simulink model "Automatisierung_Kapitel8_zustandsregler"  (R2015b)
settings: Solver=ode45  StartTime=0.0  StopTime=100  MaxStep=0.2  RelTol=1e-3
values from neighbouring files (symbols this model uses):
  Ac = [0,1,0,0;-1,-1,1,1;0,0,0,1;0.1,0.1,-0.2,-0.2]    [Automatisierung_Kapitel8.m]
  Bc = [bc,bvc]    [Automatisierung_Kapitel8.m]
  Cc = eye(4)    [Automatisierung_Kapitel8.m]
  Dc = [0,0;0,0;0,0;0,0]    [Automatisierung_Kapitel8.m]
  g = 1/((cc+dc*k)*inv(eye(4)-Ad-bd*k)*bd+dc)    [Automatisierung_Kapitel8.m]
  k = -acker(Ad,bd,pd)    [Automatisierung_Kapitel8.m]
  Ta = 2    [Automatisierung_Kapitel8.m]
settings Model: Creator=aku  LastModifiedBy=hk
settings DataIOCC: SaveFormat=Array  SignalLoggingSaveFormat=ModelDataLogs
settings OptimizationCC: BooleanDataType=off  ExpressionDepthLimit=2147483647  InitFltsAndDblsToZero=on
settings DebuggingCC: SaveWithParameterizedLinksMsg=none  UnderspecifiedInitializationDetection=Classic  MergeDetectMultiDrivingBlocksExec=none  SignalResolutionControl=TryResolveAllWithWarning  MultiTaskDSMMsg=warning  MultiTaskCondExecSysMsg=none  FcnCallInpInsideContextMsg=EnableAllAsWarning  StateNameClashWarn=warning
settings HardwareCC: ProdBitPerPointer=32  ProdLargestAtomicFloat=None  ProdIntDivRoundTo=Undefined  ProdEndianess=Unspecified  ProdWordSize=32  ProdHWDeviceType=32-bit Generic  TargetUnknown=on
settings GRTTargetCC: TargetFcnLib=ansi_tfl_tmw.mat  GeneratePreprocessorConditionals=Disable all  CombineOutputUpdateFcns=off  GRTInterface=on
settings ConfigComp: CovModelRefEnable=Off  CovSFcnEnable=off

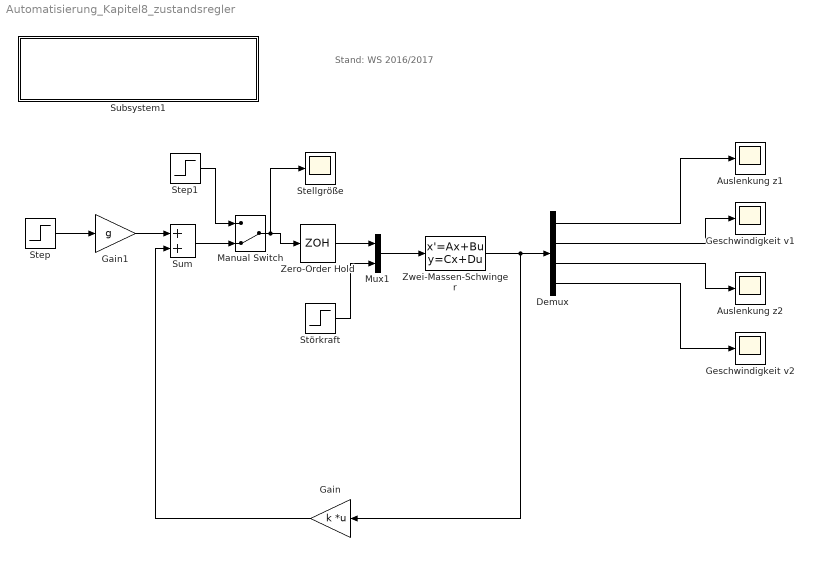
== system Automatisierung_Kapitel8_zustandsregler ==
  note: Stand: WS 2016/2017
  Auslenkung z1 : Scope
  Auslenkung z2 : Scope
  Demux : Demux
  Gain : Gain  Gain=k  Multiplication=Matrix(K*u)  SampleTime=Ta
  Gain1 : Gain  Gain=g  SampleTime=Ta
  Geschwindigkeit v1 : Scope
  Geschwindigkeit v2 : Scope
  Manual Switch : ManualSwitch  CurrentSetting=0
  Mux1 : Mux  Inputs=2
  Stellgröße : Scope
  Step : Step  Time=0  SampleTime=Ta
  Step1 : Step  Time=0  SampleTime=0
  Störkraft : Step  Time=20  SampleTime=Ta
  Subsystem1 : Subsystem
      settings: OpenFcn=Automatisierung_Kapitel8
      mask Display:
      | disp('Daten laden (Automatisierung_Kapitel8.m)\n\n');
      | disp('(mittels Doppelklick)');
  Sum : Sum
  Zero-Order Hold : ZeroOrderHold  SampleTime=Ta
  Zwei-Massen-Schwinger : StateSpace  A=Ac  B=Bc  C=Cc  D=Dc  X0=[0,0,0,0]
  wires:
  Zwei-Massen-Schwinger/1 -> Demux/1, Gain/1
  Mux1/1 -> Zwei-Massen-Schwinger/1
  Störkraft/1 -> Mux1/2
  Demux/1 -> Auslenkung z1/1
  Demux/3 -> Auslenkung z2/1
  Step/1 -> Gain1/1
  Demux/2 -> Geschwindigkeit v1/1
  Demux/4 -> Geschwindigkeit v2/1
  Gain/1 -> Sum/2
  Gain1/1 -> Sum/1
  Sum/1 -> Manual Switch/2
  Manual Switch/1 -> Stellgröße/1, Zero-Order Hold/1
  Step1/1 -> Manual Switch/1
  Zero-Order Hold/1 -> Mux1/1

== system Automatisierung_Kapitel8_zustandsregler/Subsystem1 ==
